simulink model "chapter3_PI_jd"  (R2016b)
settings: Solver=VariableStepAuto  StartTime=0.0  StopTime=10.0  RelTol=1e-3
PreLoadFcn:
  | Kp = 0.3;
  | Ki = 2;
  | Ts = 0.01;
settings Model: Creator=training-ah  LastModifiedBy=training-ah

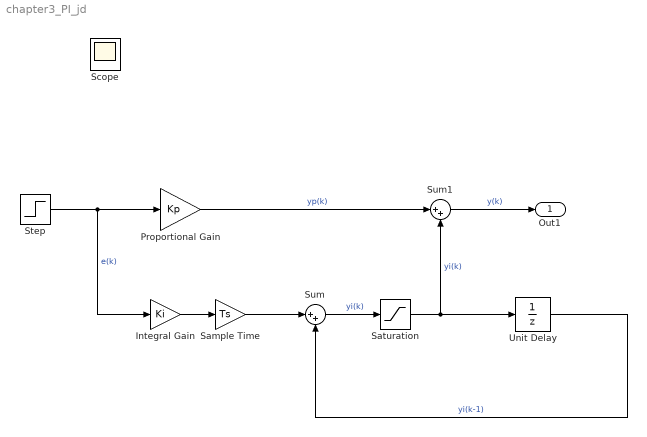
== system chapter3_PI_jd ==
  Integral Gain : Gain  Gain=Ki
  Proportional Gain : Gain  Gain=Kp
  Sample Time : Gain  Gain=Ts
  Saturation : Saturate  UpperLimit=1  LowerLimit=-1
      settings: AttributesFormatString=%<LowerLimit> <= yi(k) <= %<UpperLimit>
  Step : Step  SampleTime=Ts
  Sum : Sum  Inputs=|++
  Sum1 : Sum  Inputs=|++
  Unit Delay : UnitDelay  SampleTime=Ts
  Out1 : Outport
  Scope : Scope
  wires:
  Unit Delay/1 -> Sum/2  "yi(k-1)"
  Saturation/1 -> Sum1/2, Unit Delay/1  "yi(k)"
  Step/1 -> Integral Gain/1, Proportional Gain/1  "e(k)"
  Proportional Gain/1 -> Sum1/1  "yp(k)"
  Integral Gain/1 -> Sample Time/1
  Sample Time/1 -> Sum/1
  Sum1/1 -> Out1/1  "y(k)"
  Sum/1 -> Saturation/1  "yi(k)"
